simulink model "Kalman_test"  (R2015a)
settings: Solver=ode2  StartTime=0.0  StopTime=50  FixedStep=0.01  RelTol=1e-3
StopFcn:
  | Kalman_output
undefined symbols (not defined in the file or in its folder): sigbuilder_block
settings Model: CovModelRefEnable=off  Creator=asus  LastModifiedBy=Mattia
settings DataIOCC: SaveFormat=Dataset
settings HardwareCC: ProdBitPerPointer=64  ProdLargestAtomicFloat=Float  ProdIntDivRoundTo=Zero  ProdEndianess=LittleEndian  ProdHWDeviceType=Specified
settings GRTTargetCC: GeneratePreprocessorConditionals=Use local settings

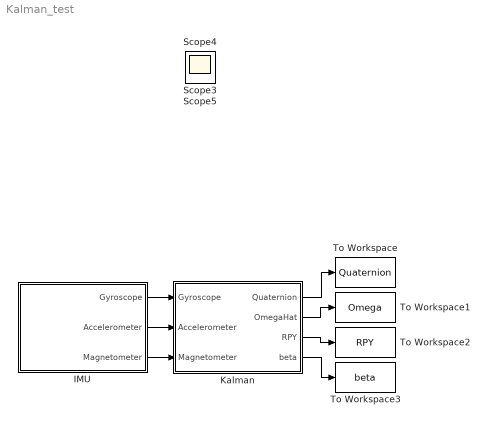
== system Kalman_test ==
  IMU : Subsystem
  Kalman : Subsystem
  To Workspace : ToWorkspace  VariableName=Quaternion  SaveFormat=Structure With Time  SampleTime=-1
  To Workspace1 : ToWorkspace  VariableName=Omega  SaveFormat=Structure With Time  SampleTime=-1
  To Workspace2 : ToWorkspace  VariableName=RPY  SaveFormat=Structure With Time  SampleTime=-1
  To Workspace3 : ToWorkspace  VariableName=beta  SaveFormat=Structure With Time  SampleTime=-1
  Scope3 : Scope
      settings: SaveName=ScopeData3
  Scope4 : Scope
      settings: SaveName=ScopeData4
  Scope5 : Scope
      settings: SaveName=ScopeData5
  wires:
  IMU/1(Gyroscope) -> Kalman/1(Gyroscope)
  IMU/2(Accelerometer) -> Kalman/2(Accelerometer)
  IMU/3("Magnetometer ") -> Kalman/3("Magnetometer ")
  Kalman/1(Quaternion) -> To Workspace/1
  Kalman/2(OmegaHat) -> To Workspace1/1
  Kalman/3(RPY) -> To Workspace2/1
  Kalman/4(beta) -> To Workspace3/1

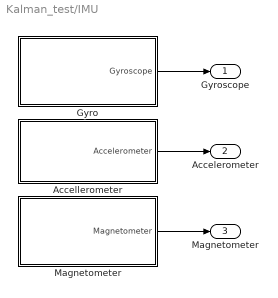
== system Kalman_test/IMU ==
  Accellerometer : Subsystem
  Gyro : Subsystem
  Magnetometer : Subsystem
  Gyroscope : Outport
  Accelerometer : Outport  Port=2
  "Magnetometer " : Outport  Port=3
  wires:
  Magnetometer/1(Magnetometer) -> "Magnetometer "/1
  Accellerometer/1(Accelerometer) -> Accelerometer/1
  Gyro/1(Gyroscope) -> Gyroscope/1

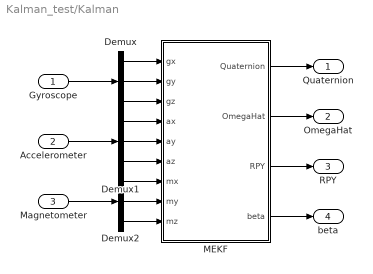
== system Kalman_test/Kalman ==
  Gyroscope : Inport
  Accelerometer : Inport  Port=2
  "Magnetometer " : Inport  Port=3
  Demux : Demux  Outputs=3
  Demux1 : Demux  Outputs=3
  Demux2 : Demux  Outputs=3
  MEKF : Subsystem
  Quaternion : Outport
  OmegaHat : Outport  Port=2
  RPY : Outport  Port=3
  beta : Outport  Port=4
  wires:
  Demux1/1 -> MEKF/4(ax)
  Demux1/2 -> MEKF/5(ay)
  Gyroscope/1 -> Demux/1
  Demux1/3 -> MEKF/6(az)
  Demux/3 -> MEKF/3(gz)
  Demux/2 -> MEKF/2(gy)
  Accelerometer/1 -> Demux1/1
  MEKF/2(OmegaHat) -> OmegaHat/1
  MEKF/1(Quaternion) -> Quaternion/1
  MEKF/3(RPY) -> RPY/1
  Demux2/1 -> MEKF/7(mx)
  "Magnetometer "/1 -> Demux2/1
  Demux2/2 -> MEKF/8(my)
  Demux2/3 -> MEKF/9(mz)
  Demux/1 -> MEKF/1(gx)
  MEKF/4("beta ") -> beta/1

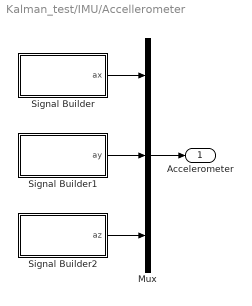
== system Kalman_test/IMU/Accellerometer ==
  Mux : Mux  Inputs=3
  Signal Builder : Subsystem  Tag=STV Subsys  LoadFcn=sigbuilder_block('load');  StartFcn=sigbuilder_block('start');  StopFcn=sigbuilder_block('stop');  ClipboardFcn=sigbuilder_block('clipboard');  mask(Sigbuilder block){}
      mask init:
      | if ~strcmp(get_param(bdroot(gcb),'SimulationStatus'),'stopped'),tuvar = sigbuilder_block('maskInit'); end
      settings: CopyFcn=sigbuilder_block('copy');  DeleteFcn=sigbuilder_block('delete');  ModelCloseFcn=sigbuilder_block('modelClose');  PreSaveFcn=sigbuilder_block('preSave');  PauseFcn=sigbuilder_block('pause');  ContinueFcn=sigbuilder_block('continue');  NameChangeFcn=sigbuilder_block('namechange');  OpenFcn=sigbuilder_block('open');  CloseFcn=sigbuilder_block('close');
      mask Display: plot(0, 0, 100, 100,[2, 2, 32, 32, 2], [68, 8, 8, 68, 68],[32, 2], [38, 38], [32, 19, 2],[53, 60, 44], [32, 17, 17, 2],[16, 16, 31, 31]);txt = getActiveGroup(gcbh);text(2, 100, txt,'verticalAlignment', 'top');
  Signal Builder1 : Subsystem  Tag=STV Subsys  LoadFcn=sigbuilder_block('load');  StartFcn=sigbuilder_block('start');  StopFcn=sigbuilder_block('stop');  ClipboardFcn=sigbuilder_block('clipboard');  mask(Sigbuilder block){}
      mask init:
      | if ~strcmp(get_param(bdroot(gcb),'SimulationStatus'),'stopped'),tuvar = sigbuilder_block('maskInit'); end
      settings: CopyFcn=sigbuilder_block('copy');  DeleteFcn=sigbuilder_block('delete');  ModelCloseFcn=sigbuilder_block('modelClose');  PreSaveFcn=sigbuilder_block('preSave');  PauseFcn=sigbuilder_block('pause');  ContinueFcn=sigbuilder_block('continue');  NameChangeFcn=sigbuilder_block('namechange');  OpenFcn=sigbuilder_block('open');  CloseFcn=sigbuilder_block('close');
      mask Display: plot(0, 0, 100, 100,[2, 2, 32, 32, 2], [68, 8, 8, 68, 68],[32, 2], [38, 38], [32, 19, 2],[53, 60, 44], [32, 17, 17, 2],[16, 16, 31, 31]);txt = getActiveGroup(gcbh);text(2, 100, txt,'verticalAlignment', 'top');
  Signal Builder2 : Subsystem  Tag=STV Subsys  LoadFcn=sigbuilder_block('load');  StartFcn=sigbuilder_block('start');  StopFcn=sigbuilder_block('stop');  ClipboardFcn=sigbuilder_block('clipboard');  mask(Sigbuilder block){}
      mask init:
      | if ~strcmp(get_param(bdroot(gcb),'SimulationStatus'),'stopped'),tuvar = sigbuilder_block('maskInit'); end
      settings: CopyFcn=sigbuilder_block('copy');  DeleteFcn=sigbuilder_block('delete');  ModelCloseFcn=sigbuilder_block('modelClose');  PreSaveFcn=sigbuilder_block('preSave');  PauseFcn=sigbuilder_block('pause');  ContinueFcn=sigbuilder_block('continue');  NameChangeFcn=sigbuilder_block('namechange');  OpenFcn=sigbuilder_block('open');  CloseFcn=sigbuilder_block('close');
      mask Display: plot(0, 0, 100, 100,[2, 2, 32, 32, 2], [68, 8, 8, 68, 68],[32, 2], [38, 38], [32, 19, 2],[53, 60, 44], [32, 17, 17, 2],[16, 16, 31, 31]);txt = getActiveGroup(gcbh);text(2, 100, txt,'verticalAlignment', 'top');
  Accelerometer : Outport
  wires:
  Mux/1 -> Accelerometer/1
  Signal Builder/1(ax) -> Mux/1
  Signal Builder1/1(ay) -> Mux/2
  Signal Builder2/1(az) -> Mux/3

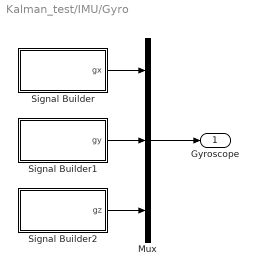
== system Kalman_test/IMU/Gyro ==
  Mux : Mux  Inputs=3
  Signal Builder : Subsystem  Tag=STV Subsys  LoadFcn=sigbuilder_block('load');  StartFcn=sigbuilder_block('start');  StopFcn=sigbuilder_block('stop');  ClipboardFcn=sigbuilder_block('clipboard');  mask(Sigbuilder block){}
      mask init:
      | if ~strcmp(get_param(bdroot(gcb),'SimulationStatus'),'stopped'),tuvar = sigbuilder_block('maskInit'); end
      settings: CopyFcn=sigbuilder_block('copy');  DeleteFcn=sigbuilder_block('delete');  ModelCloseFcn=sigbuilder_block('modelClose');  PreSaveFcn=sigbuilder_block('preSave');  PauseFcn=sigbuilder_block('pause');  ContinueFcn=sigbuilder_block('continue');  NameChangeFcn=sigbuilder_block('namechange');  OpenFcn=sigbuilder_block('open');  CloseFcn=sigbuilder_block('close');
      mask Display: plot(0, 0, 100, 100,[2, 2, 32, 32, 2], [68, 8, 8, 68, 68],[32, 2], [38, 38], [32, 19, 2],[53, 60, 44], [32, 17, 17, 2],[16, 16, 31, 31]);txt = getActiveGroup(gcbh);text(2, 100, txt,'verticalAlignment', 'top');
  Signal Builder1 : Subsystem  Tag=STV Subsys  LoadFcn=sigbuilder_block('load');  StartFcn=sigbuilder_block('start');  StopFcn=sigbuilder_block('stop');  ClipboardFcn=sigbuilder_block('clipboard');  mask(Sigbuilder block){}
      mask init:
      | if ~strcmp(get_param(bdroot(gcb),'SimulationStatus'),'stopped'),tuvar = sigbuilder_block('maskInit'); end
      settings: CopyFcn=sigbuilder_block('copy');  DeleteFcn=sigbuilder_block('delete');  ModelCloseFcn=sigbuilder_block('modelClose');  PreSaveFcn=sigbuilder_block('preSave');  PauseFcn=sigbuilder_block('pause');  ContinueFcn=sigbuilder_block('continue');  NameChangeFcn=sigbuilder_block('namechange');  OpenFcn=sigbuilder_block('open');  CloseFcn=sigbuilder_block('close');
      mask Display: plot(0, 0, 100, 100,[2, 2, 32, 32, 2], [68, 8, 8, 68, 68],[32, 2], [38, 38], [32, 19, 2],[53, 60, 44], [32, 17, 17, 2],[16, 16, 31, 31]);txt = getActiveGroup(gcbh);text(2, 100, txt,'verticalAlignment', 'top');
  Signal Builder2 : Subsystem  Tag=STV Subsys  LoadFcn=sigbuilder_block('load');  StartFcn=sigbuilder_block('start');  StopFcn=sigbuilder_block('stop');  ClipboardFcn=sigbuilder_block('clipboard');  mask(Sigbuilder block){}
      mask init:
      | if ~strcmp(get_param(bdroot(gcb),'SimulationStatus'),'stopped'),tuvar = sigbuilder_block('maskInit'); end
      settings: CopyFcn=sigbuilder_block('copy');  DeleteFcn=sigbuilder_block('delete');  ModelCloseFcn=sigbuilder_block('modelClose');  PreSaveFcn=sigbuilder_block('preSave');  PauseFcn=sigbuilder_block('pause');  ContinueFcn=sigbuilder_block('continue');  NameChangeFcn=sigbuilder_block('namechange');  OpenFcn=sigbuilder_block('open');  CloseFcn=sigbuilder_block('close');
      mask Display: plot(0, 0, 100, 100,[2, 2, 32, 32, 2], [68, 8, 8, 68, 68],[32, 2], [38, 38], [32, 19, 2],[53, 60, 44], [32, 17, 17, 2],[16, 16, 31, 31]);txt = getActiveGroup(gcbh);text(2, 100, txt,'verticalAlignment', 'top');
  Gyroscope : Outport
  wires:
  Mux/1 -> Gyroscope/1
  Signal Builder/1(gx) -> Mux/1
  Signal Builder1/1(gy) -> Mux/2
  Signal Builder2/1(gz) -> Mux/3

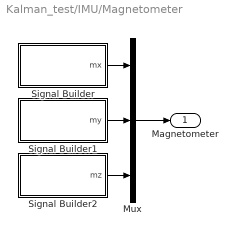
== system Kalman_test/IMU/Magnetometer ==
  Mux : Mux  Inputs=3
  Signal Builder : Subsystem  Tag=STV Subsys  LoadFcn=sigbuilder_block('load');  StartFcn=sigbuilder_block('start');  StopFcn=sigbuilder_block('stop');  ClipboardFcn=sigbuilder_block('clipboard');  mask(Sigbuilder block){}
      mask init:
      | if ~strcmp(get_param(bdroot(gcb),'SimulationStatus'),'stopped'),tuvar = sigbuilder_block('maskInit'); end
      settings: CopyFcn=sigbuilder_block('copy');  DeleteFcn=sigbuilder_block('delete');  ModelCloseFcn=sigbuilder_block('modelClose');  PreSaveFcn=sigbuilder_block('preSave');  PauseFcn=sigbuilder_block('pause');  ContinueFcn=sigbuilder_block('continue');  NameChangeFcn=sigbuilder_block('namechange');  OpenFcn=sigbuilder_block('open');  CloseFcn=sigbuilder_block('close');
      mask Display: plot(0, 0, 100, 100,[2, 2, 32, 32, 2], [68, 8, 8, 68, 68],[32, 2], [38, 38], [32, 19, 2],[53, 60, 44], [32, 17, 17, 2],[16, 16, 31, 31]);txt = getActiveGroup(gcbh);text(2, 100, txt,'verticalAlignment', 'top');
  Signal Builder1 : Subsystem  Tag=STV Subsys  LoadFcn=sigbuilder_block('load');  StartFcn=sigbuilder_block('start');  StopFcn=sigbuilder_block('stop');  ClipboardFcn=sigbuilder_block('clipboard');  mask(Sigbuilder block){}
      mask init:
      | if ~strcmp(get_param(bdroot(gcb),'SimulationStatus'),'stopped'),tuvar = sigbuilder_block('maskInit'); end
      settings: CopyFcn=sigbuilder_block('copy');  DeleteFcn=sigbuilder_block('delete');  ModelCloseFcn=sigbuilder_block('modelClose');  PreSaveFcn=sigbuilder_block('preSave');  PauseFcn=sigbuilder_block('pause');  ContinueFcn=sigbuilder_block('continue');  NameChangeFcn=sigbuilder_block('namechange');  OpenFcn=sigbuilder_block('open');  CloseFcn=sigbuilder_block('close');
      mask Display: plot(0, 0, 100, 100,[2, 2, 32, 32, 2], [68, 8, 8, 68, 68],[32, 2], [38, 38], [32, 19, 2],[53, 60, 44], [32, 17, 17, 2],[16, 16, 31, 31]);txt = getActiveGroup(gcbh);text(2, 100, txt,'verticalAlignment', 'top');
  Signal Builder2 : Subsystem  Tag=STV Subsys  LoadFcn=sigbuilder_block('load');  StartFcn=sigbuilder_block('start');  StopFcn=sigbuilder_block('stop');  ClipboardFcn=sigbuilder_block('clipboard');  mask(Sigbuilder block){}
      mask init:
      | if ~strcmp(get_param(bdroot(gcb),'SimulationStatus'),'stopped'),tuvar = sigbuilder_block('maskInit'); end
      settings: CopyFcn=sigbuilder_block('copy');  DeleteFcn=sigbuilder_block('delete');  ModelCloseFcn=sigbuilder_block('modelClose');  PreSaveFcn=sigbuilder_block('preSave');  PauseFcn=sigbuilder_block('pause');  ContinueFcn=sigbuilder_block('continue');  NameChangeFcn=sigbuilder_block('namechange');  OpenFcn=sigbuilder_block('open');  CloseFcn=sigbuilder_block('close');
      mask Display: plot(0, 0, 100, 100,[2, 2, 32, 32, 2], [68, 8, 8, 68, 68],[32, 2], [38, 38], [32, 19, 2],[53, 60, 44], [32, 17, 17, 2],[16, 16, 31, 31]);txt = getActiveGroup(gcbh);text(2, 100, txt,'verticalAlignment', 'top');
  Magnetometer : Outport
  wires:
  Mux/1 -> Magnetometer/1
  Signal Builder/1(mx) -> Mux/1
  Signal Builder1/1(my) -> Mux/2
  Signal Builder2/1(mz) -> Mux/3

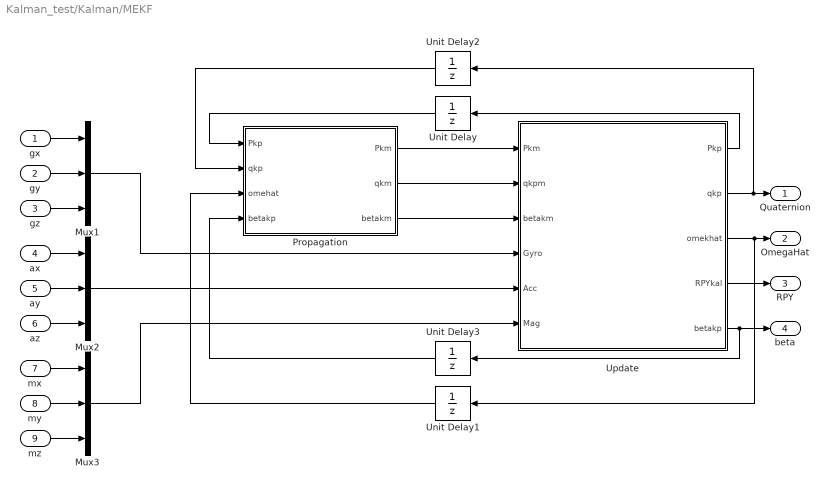
== system Kalman_test/Kalman/MEKF ==
  gx : Inport
  gy : Inport  Port=2
  gz : Inport  Port=3
  ax : Inport  Port=4
  ay : Inport  Port=5
  az : Inport  Port=6
  mx : Inport  Port=7
  my : Inport  Port=8
  mz : Inport  Port=9
  Mux1 : Mux  Inputs=3
  Mux2 : Mux  Inputs=3
  Mux3 : Mux  Inputs=3
  "Propagation " : MATLAB Function  TreatAsAtomicUnit=on
  Unit Delay : UnitDelay  InitialCondition=(1e-6)*[1 0 0 0 0 0; 0 1 0 0 0 0; 0 0 1 0 0 0; 0 0 0 1 0 0; 0 0 0 0 1 0; 0 0 0 0 0 1]  SampleTime=-1
  Unit Delay1 : UnitDelay  InitialCondition=0.00001*[1 1 1]'  SampleTime=-1
  Unit Delay2 : UnitDelay  InitialCondition=[0 0 0 1]'  SampleTime=-1
  Unit Delay3 : UnitDelay  InitialCondition=0.00001*[1 1 1]'  SampleTime=-1
  Update : MATLAB Function  TreatAsAtomicUnit=on
  Quaternion : Outport
  OmegaHat : Outport  Port=2
  RPY : Outport  Port=3
  "beta " : Outport  Port=4
  wires:
  Update/1(Pkp) -> Unit Delay/1
  Update/3(omekhat) -> Unit Delay1/1, OmegaHat/1
  Unit Delay1/1 -> "Propagation "/3(omehat)
  Unit Delay/1 -> "Propagation "/1(Pkp)
  "Propagation "/1(Pkm) -> Update/1(Pkm)
  gx/1 -> Mux1/1
  gy/1 -> Mux1/2
  ax/1 -> Mux2/1
  mx/1 -> Mux3/1
  az/1 -> Mux2/3
  Update/2(qkp) -> Unit Delay2/1, Quaternion/1
  Update/5(betakp) -> Unit Delay3/1, "beta "/1
  gz/1 -> Mux1/3
  ay/1 -> Mux2/2
  Unit Delay2/1 -> "Propagation "/2(qkp)
  "Propagation "/2(qkm) -> Update/2(qkpm)
  mz/1 -> Mux3/3
  my/1 -> Mux3/2
  Mux1/1 -> Update/4(Gyro)
  Mux2/1 -> Update/5(Acc)
  Mux3/1 -> Update/6(Mag)
  Unit Delay3/1 -> "Propagation "/4(betakp)
  Update/4(RPYkal) -> RPY/1
  "Propagation "/3(betakm) -> Update/3(betakm)

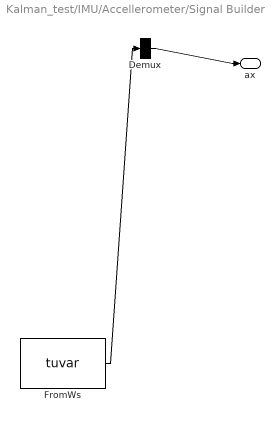
== system Kalman_test/IMU/Accellerometer/Signal Builder ==
  Demux : Demux  Tag=STV Demux  Outputs=1
  FromWs : FromWorkspace  Tag=STV FromWs  VariableName=tuvar  SampleTime=0
      SigBuilderData=|
      | dataSet.timeRange = [0 49.99]
      | dataSet.name = 'Group 1'
      | sbobj.Name = 'Signal Builder'
      | sbobj.Groups.Name = 'Group 1'
      | sbobj.Groups.Signals.Name = 'ax'
      | sbobj.Groups.Signals.XData = [0 0.01 0.02 0.03 0.04 0.05 0.06 0.07 0.08 0.09 0.1 0.11 ... (5000 elements, 1x5000)]
      | sbobj.Groups.Signals.YData = [0.1132 0.1038 0.0004 0.0474 0.2636 -0.2534 0.1414 0.2636 -0.338 0.3952 0.0474 -0.3286 ... (5000 elements, 1x5000)]
      | sbobj.Groups.TimeRange = [0 49.99]
  ax : Outport  Tag=STV Outport
  wires:
  FromWs/1 -> Demux/1
  Demux/1 -> ax/1

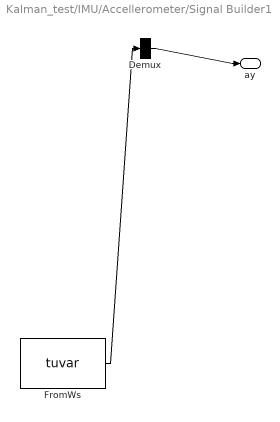
== system Kalman_test/IMU/Accellerometer/Signal Builder1 ==
  Demux : Demux  Tag=STV Demux  Outputs=1
  FromWs : FromWorkspace  Tag=STV FromWs  VariableName=tuvar  SampleTime=0
      SigBuilderData=|
      | dataSet.timeRange = [0 49.99]
      | dataSet.name = 'Group 1'
      | sbobj.Name = 'Signal Builder'
      | sbobj.Groups.Name = 'Group 1'
      | sbobj.Groups.Signals.Name = 'ay'
      | sbobj.Groups.Signals.XData = [0 0.01 0.02 0.03 0.04 0.05 0.06 0.07 0.08 0.09 0.1 0.11 ... (5000 elements, 1x5000)]
      | sbobj.Groups.Signals.YData = [0.0346 -0.1286 -0.0134 -0.071 -0.0902 0.0154 -0.0326 -0.2342 0.1018 -0.0518 -0.2726 0.2554 ... (5000 elements, 1x5000)]
      | sbobj.Groups.TimeRange = [0 49.99]
  ay : Outport  Tag=STV Outport
  wires:
  FromWs/1 -> Demux/1
  Demux/1 -> ay/1

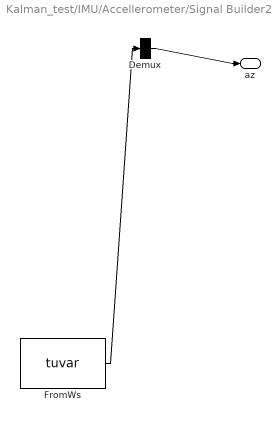
== system Kalman_test/IMU/Accellerometer/Signal Builder2 ==
  Demux : Demux  Tag=STV Demux  Outputs=1
  FromWs : FromWorkspace  Tag=STV FromWs  VariableName=tuvar  SampleTime=0
      SigBuilderData=|
      | dataSet.timeRange = [0 49.99]
      | dataSet.name = 'Group 1'
      | sbobj.Name = 'Signal Builder'
      | sbobj.Groups.Name = 'Group 1'
      | sbobj.Groups.Signals.Name = 'az'
      | sbobj.Groups.Signals.XData = [0 0.01 0.02 0.03 0.04 0.05 0.06 0.07 0.08 0.09 0.1 0.11 ... (5000 elements, 1x5000)]
      | sbobj.Groups.Signals.YData = [9.6294 9.8967 9.6591 9.7482 9.8076 9.6789 9.7284 9.8868 9.5502 10.0353 9.5898 9.6393 ... (5000 elements, 1x5000)]
      | sbobj.Groups.TimeRange = [0 49.99]
  az : Outport  Tag=STV Outport
  wires:
  FromWs/1 -> Demux/1
  Demux/1 -> az/1

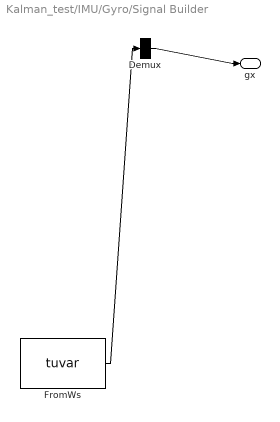
== system Kalman_test/IMU/Gyro/Signal Builder ==
  Demux : Demux  Tag=STV Demux  Outputs=1
  FromWs : FromWorkspace  Tag=STV FromWs  VariableName=tuvar  SampleTime=0
      SigBuilderData=|
      | dataSet.timeRange = [0 49.99]
      | dataSet.name = 'Group 1'
      | sbobj.Name = 'Signal Builder'
      | sbobj.Groups.Name = 'Group 1'
      | sbobj.Groups.Signals.Name = 'gx'
      | sbobj.Groups.Signals.XData = [0 0.01 0.02 0.03 0.04 0.05 0.06 0.07 0.08 0.09 0.1 0.11 ... (5000 elements, 1x5000)]
      | sbobj.Groups.Signals.YData = [0.0248358 -0.0236742 0.0172458 -0.0117942 0.0043758 0.0004158 -0.0045342 -0.0022242 0.0007458 0.0040458 -0.0207042 0.0284658 ... (5000 elements, 1x5000)]
      | sbobj.Groups.TimeRange = [0 49.99]
  gx : Outport  Tag=STV Outport
  wires:
  FromWs/1 -> Demux/1
  Demux/1 -> gx/1

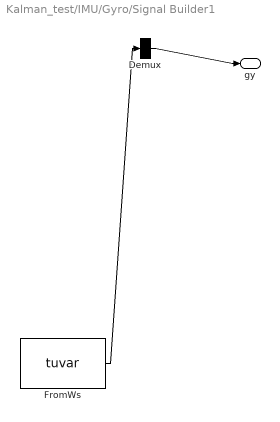
== system Kalman_test/IMU/Gyro/Signal Builder1 ==
  Demux : Demux  Tag=STV Demux  Outputs=1
  FromWs : FromWorkspace  Tag=STV FromWs  VariableName=tuvar  SampleTime=0
      SigBuilderData=|
      | dataSet.timeRange = [0 49.99]
      | dataSet.name = 'Group 1'
      | sbobj.Name = 'Signal Builder'
      | sbobj.Groups.Name = 'Group 1'
      | sbobj.Groups.Signals.Name = 'gy'
      | sbobj.Groups.Signals.XData = [0 0.01 0.02 0.03 0.04 0.05 0.06 0.07 0.08 0.09 0.1 0.11 ... (5000 elements, 1x5000)]
      | sbobj.Groups.Signals.YData = [-0.0221661 0.0187539 0.0019239 -0.0238161 0.0085239 0.0266739 -0.0521961 0.0600039 -0.0446061 -0.0096261 0.0765039 -0.0851961 ... (5000 elements, 1x5000)]
      | sbobj.Groups.TimeRange = [0 49.99]
  gy : Outport  Tag=STV Outport
  wires:
  FromWs/1 -> Demux/1
  Demux/1 -> gy/1

== system Kalman_test/IMU/Gyro/Signal Builder2 ==
  Demux : Demux  Tag=STV Demux  Outputs=1
  FromWs : FromWorkspace  Tag=STV FromWs  VariableName=tuvar  SampleTime=0
      SigBuilderData=|
      | dataSet.timeRange = [0 49.99]
      | dataSet.name = 'Group 1'
      | sbobj.Name = 'Signal Builder'
      | sbobj.Groups.Name = 'Group 1'
      | sbobj.Groups.Signals.Name = 'gz'
      | sbobj.Groups.Signals.XData = [0 0.01 0.02 0.03 0.04 0.05 0.06 0.07 0.08 0.09 0.1 0.11 ... (5000 elements, 1x5000)]
      | sbobj.Groups.Signals.YData = [0.0178436 -0.0010664 -0.0212164 0.0336536 -0.0243164 -0.0125364 0.0389236 -0.0295864 -0.0178064 0.0584536 -0.0757764 0.0534936 ... (5000 elements, 1x5000)]
      | sbobj.Groups.TimeRange = [0 49.99]
  gz : Outport  Tag=STV Outport
  wires:
  FromWs/1 -> Demux/1
  Demux/1 -> gz/1

== system Kalman_test/IMU/Magnetometer/Signal Builder ==
  Demux : Demux  Tag=STV Demux  Outputs=1
  FromWs : FromWorkspace  Tag=STV FromWs  VariableName=tuvar  SampleTime=0
      SigBuilderData=|
      | dataSet.timeRange = [0 49.99]
      | dataSet.name = 'Group 1'
      | sbobj.Name = 'Signal Builder'
      | sbobj.Groups.Name = 'Group 1'
      | sbobj.Groups.Signals.Name = 'mx'
      | sbobj.Groups.Signals.XData = [0 0.01 0.02 0.03 0.04 0.05 0.06 0.07 0.08 0.09 0.1 0.11 ... (5000 elements, 1x5000)]
      | sbobj.Groups.Signals.YData = [-0.1656 -0.16 -0.16 -0.1712 -0.1796 -0.1656 -0.1768 -0.1796 -0.1796 -0.174 -0.1768 -0.174 ... (5000 elements, 1x5000)]
      | sbobj.Groups.TimeRange = [0 49.99]
  mx : Outport  Tag=STV Outport
  wires:
  FromWs/1 -> Demux/1
  Demux/1 -> mx/1

== system Kalman_test/IMU/Magnetometer/Signal Builder1 ==
  Demux : Demux  Tag=STV Demux  Outputs=1
  FromWs : FromWorkspace  Tag=STV FromWs  VariableName=tuvar  SampleTime=0
      SigBuilderData=|
      | dataSet.timeRange = [0 49.99]
      | dataSet.name = 'Group 1'
      | sbobj.Name = 'Signal Builder'
      | sbobj.Groups.Name = 'Group 1'
      | sbobj.Groups.Signals.Name = 'my'
      | sbobj.Groups.Signals.XData = [0 0.01 0.02 0.03 0.04 0.05 0.06 0.07 0.08 0.09 0.1 0.11 ... (5000 elements, 1x5000)]
      | sbobj.Groups.Signals.YData = [-0.3236 -0.3292 -0.332 -0.3292 -0.3376 -0.3348 -0.3376 -0.3376 -0.3376 -0.3348 -0.3292 -0.3348 ... (5000 elements, 1x5000)]
      | sbobj.Groups.TimeRange = [0 49.99]
  my : Outport  Tag=STV Outport
  wires:
  FromWs/1 -> Demux/1
  Demux/1 -> my/1

== system Kalman_test/IMU/Magnetometer/Signal Builder2 ==
  Demux : Demux  Tag=STV Demux  Outputs=1
  FromWs : FromWorkspace  Tag=STV FromWs  VariableName=tuvar  SampleTime=0
      SigBuilderData=|
      | dataSet.timeRange = [0 49.99]
      | dataSet.name = 'Group 1'
      | sbobj.Name = 'Signal Builder'
      | sbobj.Groups.Name = 'Group 1'
      | sbobj.Groups.Signals.Name = 'mz'
      | sbobj.Groups.Signals.XData = [0 0.01 0.02 0.03 0.04 0.05 0.06 0.07 0.08 0.09 0.1 0.11 ... (5000 elements, 1x5000)]
      | sbobj.Groups.Signals.YData = [-0.058 -0.055 -0.046 -0.037 -0.04 -0.052 -0.049 -0.052 -0.052 -0.055 -0.04 -0.043 ... (5000 elements, 1x5000)]
      | sbobj.Groups.TimeRange = [0 49.99]
  mz : Outport  Tag=STV Outport
  wires:
  FromWs/1 -> Demux/1
  Demux/1 -> mz/1

== matlab function Kalman_test/Kalman/MEKF/Update ==
  data Pkm settings: description=A-priori state estimate.
  data qkpm settings: description=A-priori covariance estimate.
  data betakm settings: description=Measurements from the sensors.
  data Pkp settings: description=Corrected state estimate.
  data omekhat settings: description=Corrected covariance estimate.
  data: Pkm input; qkpm input; betakm input; Gyro input; Pkp output; qkp output; omekhat output; RPYkal output; Acc input; Mag input; betakp output
%% EKF - Update           %
% Author: Mattia Giurato  %
% Last review: 2016/03/15 %
%%%%%%%%%%%%%%%%%%%%%%%%%%%
function [Pkp,qkp,omekhat,RPYkal,betakp] = Update(Pkm,qkpm,betakm,Gyro,Acc,Mag)
gx = Gyro(1);
gy = Gyro(2);
gz = Gyro(3);
ax = Acc(1);
ay = Acc(2);
az = Acc(3);
mx = Mag(1);
my = Mag(2);
mz = Mag(3);
Gyroscope = [gx gy gz]';
Accelerometer = [ax ay az]';
Magnetometer = [mx my mz]';

% Usefull values
sigma_acc = diag([0.77418 0.66936 0.71485]);
sigma_mag = 300*diag([0.053667 0.034382 0.071054]);
I3 = [1 0 0; 0 1 0; 0 0 1];
I6 = [1 0 0 0 0 0; 0 1 0 0 0 0; 0 0 1 0 0 0; 0 0 0 1 0 0; 0 0 0 0 1 0; 0 0 0 0 0 1];
O3 = [0 0 0; 0 0 0; 0 0 0];

% Normalise accelerometer measurement
% if(norm(Accelerometer) == 0), return; end % handle NaN
b_acc = Accelerometer / sqrt(ax^2 + ay^2 + az^2); % normalise magnitude

% Normalise magnetometer measurement
% if(norm(Magnetometer) == 0), return; end % handle NaN
b_mag = Magnetometer / sqrt(mx^2 + my^2 + mz^2); % normalise magnitude

%% Propagated value from previous step
deltaXkm = zeros(6,1);

%% Accelerometer and Magnetometer correction
% Compute attitude matrix
ro = [qkpm(1) ;
      qkpm(2) ;
      qkpm(3)];
q_4 = qkpm(4);
rox = [   0   -ro(3)  ro(2) ;
         ro(3)  0    -ro(1) ;
        -ro(2) ro(1)   0   ];
norm_ro_sq = ro(1)^2 + ro(2)^2 + ro(3)^2;
Aqkm = (q_4^2 - norm_ro_sq)*I3 + 2*(ro*ro') - 2*q_4*rox;
% Reference direction of Earth's gravitational field
r_acc = [0 ;
         0 ;
         1];
Aqmr = Aqkm*r_acc;
b = b_acc;
R = sigma_acc^2*I3;

% Sensitivity Matrix
Aqmrx = [   0     -Aqmr(3)  Aqmr(2) ;
          Aqmr(3)    0     -Aqmr(1) ;
         -Aqmr(2)  Aqmr(1)    0    ];
Hk = [Aqmrx O3];

% Gain
Kk = (Pkm*Hk')/(Hk*Pkm*Hk' + R);

% Update Covariance
Pkp = (I6 - Kk*Hk)*Pkm*(I6 - Kk*Hk)' + Kk*R*Kk';

% Update state
epk = b - Aqmr; %residual
yk = epk - Hk*deltaXkm;
deltaXkp = (deltaXkm + Kk*yk);

Pkm = Pkp;
deltaXkm = deltaXkp;

% Reference direction of Earth's magnetic feild
h = Aqkm*Magnetometer;
norm_h = sqrt(h(1)^2 + h(2)^2);
r_mag = [norm_h ;
           0    ;
          h(3) ];
Aqmr = Aqkm*r_mag;
b = b_mag;
R = sigma_mag^2*I3;

% Sensitivity Matrix
Aqmrx = [      0   -Aqmr(3)  Aqmr(2) ;
           Aqmr(3)    0     -Aqmr(1) ;
          -Aqmr(2)  Aqmr(1)    0    ];
Hk = [Aqmrx O3];

% Gain
Kk = (Pkm*Hk')/(Hk*Pkm*Hk' + R);

% Update Covariance
Pkp = (I6 - Kk*Hk)*Pkm*(I6 - Kk*Hk)' + Kk*R*Kk';

% Update state
epk = b - Aqmr; %residual
yk = epk - Hk*deltaXkm;
deltaXkp = (deltaXkm + Kk*yk);

% Update quaternion
dalphak = deltaXkp(1:3,1);
norm_dalphak_sq = dalphak(1)^2 + dalphak(2)^2 + dalphak(3)^2;
dq = (1/sqrt(4+norm_dalphak_sq))*[dalphak' 2]';
qkp = [dq(4)*ro + q_4*dq(1:3,1)-cross(dq(1:3,1),ro) ;
               dq(4)*q_4 - dot(dq(1:3,1),ro)       ];

% Update biases
deltaBeta = deltaXkp(4:6,1);
betakp = betakm + deltaBeta;
  
%% Depolarize gyroscope measurement
omekhat = Gyroscope - betakp;

%% Convert Quaternion into RPY
a1 = 2.*(qkp(1).*qkp(2) + qkp(4).*qkp(3));
a2 = qkp(4).^2 + qkp(1).^2 - qkp(2).^2 - qkp(3).^2;
b = -2.*(qkp(1).*qkp(3) - qkp(4).*qkp(2));
c1 = 2.*(qkp(2).*qkp(3) + qkp(4).*qkp(1));
c2 = qkp(4).^2 - qkp(1).^2 - qkp(2).^2 + qkp(3).^2;

Yy = atan2( a1, a2 );
Pp = asin( b );
Rr = atan2( c1, c2 );

RPYkal = [Rr -Pp -Yy]';

== matlab function Kalman_test/Kalman/MEKF/Propagation  ==
  data Pkp settings: description=Control signal at the previous step.
  data qkp settings: description=Covariance estimate at the previous step.
  data Pkm settings: description=A-priori covariance estimate.
  data qkm settings: description=A-priori state estimate.
  data: Pkp input; qkp input; Pkm output; qkm output; omehat input; betakp input; betakm output
%% EKF - Propagation      %
% Author: Mattia Giurato  %
% Last review: 2016/03/15 %
%%%%%%%%%%%%%%%%%%%%%%%%%%%
function [Pkm,qkm,betakm] = Propagation(Pkp,qkp,omehat,betakp)
%% Usefull values
sigma_u = diag([0.13807 0.11053 0.063833/10])/100;
sigma_v = diag([0.00001 0.00001 0.05]);
dt = 0.01;
I3 = [1 0 0; 0 1 0; 0 0 1];
O3 = [0 0 0; 0 0 0; 0 0 0];

%% Quaternion propagation
omex = [     0      -omehat(3)  omehat(2) ;
         omehat(3)      0      -omehat(1) ;
        -omehat(2)  omehat(1)      0     ];
Omega = [ -omex   omehat ;
         -omehat'     0 ];
qt = (eye(4) + .5*Omega*dt)*qkp;
qkm = qt / sqrt(qt(1)^2+qt(2)^2+qt(3)^2+qt(4)^2);

%% Bias propagation
betakm = betakp; 

%% Covariance equation propagation
% omekhatx = [     0      -omehat(3)  omehat(2) ;
%              omehat(3)     0       -omehat(1) ;
%             -omehat(2)  omehat(1)      0     ];
% nomehat = sqrt(omehat(1)^2+omehat(2)^2+omehat(3)^2);
% Phi1 = I3 - omekhatx*sin(nomehat*dt)/nomehat + omekhatx*omekhatx*(1 - cos(nomehat*dt))/(nomehat^2);
% Phi2 = omekhatx*(1 - cos(nomehat*dt))/(nomehat^2) - I3*dt - omekhatx*omekhatx*(nomehat*dt - sin(nomehat*dt))/(nomehat^3);
Phi1 = I3;
Phi2 = -I3*dt;
Phi = [Phi1 Phi2 ;
        O3   I3 ];
gamma = [-I3 O3 ;
          O3 I3];
Q = [(sigma_v^2*dt + 1/3*sigma_u^2*dt^3)*I3 (.5*sigma_u^2*dt^2)*I3 ;
             (.5*sigma_u^2*dt^2)*I3            (sigma_u^2*dt)*I3  ];
Pkm = Phi*Pkp*Phi' + gamma*Q*gamma';
